simulink model "five_model"  (Simulink 7.9)
settings: Solver=ode3  StartTime=0.0  StopTime=5  FixedStep=0.005  RelTol=1e-3
values from neighbouring files (symbols this model uses):
  a = -1.0    (= -1)    [five_para.m]
  Ah = 0.234    [five_para.m]
  Ak = 0.227    [five_para.m]
  b = -2.0    (= -2)    [five_para.m]
  c = 0.23    [five_para.m]
  pf = 0.1786    [five_para.m]
  ph = 0.1786    [five_para.m]
  pw = 0.1786    [five_para.m]
  Ta = 0.38    [five_para.m]
  Tr = 0.04    [five_para.m]
  u0 = 0.1*rand(4,5)    [five_para.m]
  W = [0 -1 1 -1 -1; -1 0 -1 1 -1; 1 -1 0 -1 1; -1 1 -1 0 1;-1 -1 1 1 0]    [five_para.m]
settings Model: Creator=dede  LastModifiedBy=dede

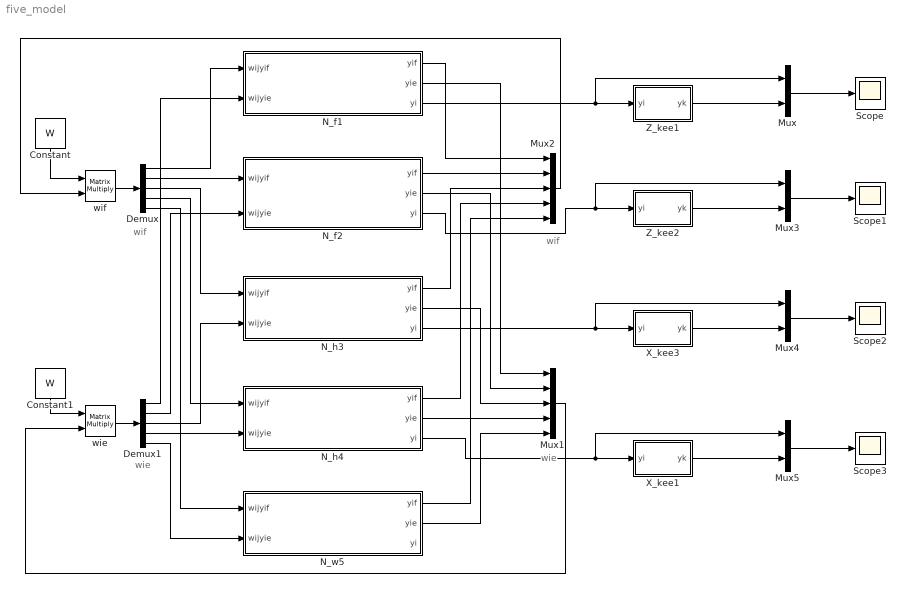
== system five_model ==
  note: wif
  note: wie
  note: wif
  note: wie
  Constant : Constant  Value=W
  Constant1 : Constant  Value=W
  Demux : Demux  Outputs=5
  Demux1 : Demux  Outputs=5
  Mux{,3..5} (4 alike) : Mux  Inputs=2
  Mux1 : Mux  Inputs=5
  Mux2 : Mux  Inputs=5
  N_f1 : Subsystem
  N_f2 : Subsystem
  N_h3 : Subsystem
  N_h4 : Subsystem
  N_w5 : Subsystem
  Scope{,1..3} (4 alike) : Scope
      Scope2 settings: SaveName=ScopeData2
      Scope3 settings: SaveName=ScopeData3
  X_kee1 : Subsystem
  X_kee3 : Subsystem
  Z_kee1 : Subsystem
  Z_kee2 : Subsystem
  wie : Product  Multiplication=Matrix(*)  RndMeth=Zero
  wif : Product  Multiplication=Matrix(*)  RndMeth=Zero
  wires:
  N_f1/1(yif) -> Mux2/1
  N_f2/1(yif) -> Mux2/2
  N_h3/1(yif) -> Mux2/3
  N_h4/1(yif) -> Mux2/4
  N_w5/1(yif) -> Mux2/5
  N_f1/2(yie) -> Mux1/1
  N_f2/2(yie) -> Mux1/2
  N_h3/2(yie) -> Mux1/3
  N_h4/2(yie) -> Mux1/4
  N_w5/2(yie) -> Mux1/5
  Demux/1 -> N_f1/1(wijyif)
  Demux/2 -> N_f2/1(wijyif)
  Demux/3 -> N_h3/1(wijyif)
  Demux/4 -> N_h4/1(wijyif)
  Demux/5 -> N_w5/1(wijyif)
  Demux1/1 -> N_f1/2(wijyie)
  Demux1/2 -> N_f2/2(wijyie)
  Demux1/3 -> N_h3/2(wijyie)
  Demux1/4 -> N_h4/2(wijyie)
  Demux1/5 -> N_w5/2(wijyie)
  Mux2/1 -> wif/2
  Constant/1 -> wif/1
  Mux1/1 -> wie/2
  Constant1/1 -> wie/1
  wie/1 -> Demux1/1
  wif/1 -> Demux/1
  N_f1/3(yi) -> Z_kee1/1(yi), Mux/1
  N_f2/3(yi) -> Z_kee2/1(yi), Mux3/1
  N_h3/3(yi) -> X_kee3/1(yi), Mux4/1
  N_h4/3(yi) -> X_kee1/1(yi), Mux5/1
  Z_kee1/1(yk) -> Mux/2
  Mux/1 -> Scope/1
  Z_kee2/1(yk) -> Mux3/2
  Mux3/1 -> Scope1/1
  X_kee3/1(yk) -> Mux4/2
  Mux4/1 -> Scope2/1
  Mux5/1 -> Scope3/1
  X_kee1/1(yk) -> Mux5/2

== system five_model/N_f1 ==
  wijyif : Inport
  wijyie : Inport  Port=2
  Gain : Gain  Gain=pf
  N_e1 : Subsystem
  N_f1 : Subsystem
  Sum : Sum  Inputs=+-
  yif : Outport
  yie : Outport  Port=2
  yi : Outport  Port=3
  wires:
  N_f1/2(yif) -> N_e1/1(yif), yif/1
  N_e1/2(yie) -> N_f1/1(yie), yie/1
  wijyif/1 -> N_f1/2(wijyif)
  wijyie/1 -> N_e1/2(wijyie)
  N_f1/1(uif) -> Sum/1
  N_e1/1(uie) -> Sum/2
  Sum/1 -> Gain/1
  Gain/1 -> yi/1

== system five_model/N_f2 ==
  wijyif : Inport
  wijyie : Inport  Port=2
  Gain : Gain  Gain=pf
  N_e1 : Subsystem
  N_f1 : Subsystem
  Sum : Sum  Inputs=+-
  yif : Outport
  yie : Outport  Port=2
  yi : Outport  Port=3
  wires:
  Gain/1 -> yi/1
  Sum/1 -> Gain/1
  N_e1/1(uie) -> Sum/2
  N_f1/1(uif) -> Sum/1
  wijyie/1 -> N_e1/2(wijyie)
  wijyif/1 -> N_f1/2(wijyif)
  N_e1/2(yie) -> yie/1, N_f1/1(yie)
  N_f1/2(yif) -> yif/1, N_e1/1(yif)

== system five_model/N_h3 ==
  wijyif : Inport
  wijyie : Inport  Port=2
  Gain : Gain  Gain=ph
  N_e1 : Subsystem
  N_f1 : Subsystem
  Sum : Sum  Inputs=+-
  yif : Outport
  yie : Outport  Port=2
  yi : Outport  Port=3
  wires:
  N_f1/2(yif) -> N_e1/1(yif), yif/1
  N_e1/2(yie) -> N_f1/1(yie), yie/1
  wijyif/1 -> N_f1/2(wijyif)
  wijyie/1 -> N_e1/2(wijyie)
  N_f1/1(uif) -> Sum/1
  N_e1/1(uie) -> Sum/2
  Sum/1 -> Gain/1
  Gain/1 -> yi/1

== system five_model/N_h4 ==
  wijyif : Inport
  wijyie : Inport  Port=2
  Gain : Gain  Gain=ph
  N_e1 : Subsystem
  N_f1 : Subsystem
  Sum : Sum  Inputs=+-
  yif : Outport
  yie : Outport  Port=2
  yi : Outport  Port=3
  wires:
  Gain/1 -> yi/1
  Sum/1 -> Gain/1
  N_e1/1(uie) -> Sum/2
  N_f1/1(uif) -> Sum/1
  wijyie/1 -> N_e1/2(wijyie)
  wijyif/1 -> N_f1/2(wijyif)
  N_e1/2(yie) -> yie/1, N_f1/1(yie)
  N_f1/2(yif) -> yif/1, N_e1/1(yif)

== system five_model/N_w5 ==
  wijyif : Inport
  wijyie : Inport  Port=2
  Gain : Gain  Gain=pw
  N_e1 : Subsystem
  N_f1 : Subsystem
  Sum : Sum  Inputs=+-
  yif : Outport
  yie : Outport  Port=2
  yi : Outport  Port=3
  wires:
  N_f1/2(yif) -> N_e1/1(yif), yif/1
  N_e1/2(yie) -> N_f1/1(yie), yie/1
  wijyif/1 -> N_f1/2(wijyif)
  wijyie/1 -> N_e1/2(wijyie)
  N_f1/1(uif) -> Sum/1
  N_e1/1(uie) -> Sum/2
  Sum/1 -> Gain/1
  Gain/1 -> yi/1

== system five_model/X_kee1 ==
  yi : Inport
  Constant2 : Constant  Value=0
  Derivative : Derivative
  Subsystem : Subsystem
  Switch : Switch
  yk : Outport
  wires:
  Switch/1 -> yk/1
  Subsystem/1(Out1) -> Switch/1
  Derivative/1 -> Switch/2
  yi/1 -> Subsystem/1(In1), Derivative/1
  Constant2/1 -> Switch/3

== system five_model/X_kee3 ==
  yi : Inport
  Constant2 : Constant  Value=0
  Derivative : Derivative
  Subsystem : Subsystem
  Switch : Switch
  yk : Outport
  wires:
  Constant2/1 -> Switch/3
  yi/1 -> Derivative/1, Subsystem/1(In1)
  Derivative/1 -> Switch/2
  Subsystem/1(Out1) -> Switch/1
  Switch/1 -> yk/1

== system five_model/Z_kee1 ==
  yi : Inport
  Constant2 : Constant  Value=0
  Derivative : Derivative
  Subsystem : Subsystem
  Switch : Switch
  yk : Outport
  wires:
  Constant2/1 -> Switch/3
  yi/1 -> Derivative/1, Subsystem/1(In1)
  Derivative/1 -> Switch/2
  Subsystem/1(Out1) -> Switch/1
  Switch/1 -> yk/1

== system five_model/Z_kee2 ==
  yi : Inport
  Constant2 : Constant  Value=0
  Derivative : Derivative
  Subsystem : Subsystem
  Switch : Switch
  yk : Outport
  wires:
  Switch/1 -> yk/1
  Subsystem/1(Out1) -> Switch/1
  Derivative/1 -> Switch/2
  yi/1 -> Subsystem/1(In1), Derivative/1
  Constant2/1 -> Switch/3

== system five_model/N_f1/N_e1 ==
  yif : Inport
  wijyie : Inport  Port=2
  Constant : Constant  Value=0
  uie0 : Subsystem
  vie : Subsystem
  yie0 : Switch
  uie : Outport
  yie : Outport  Port=2
  wires:
  vie/1(vie) -> uie0/1(vie)
  yif/1 -> uie0/2(yif)
  wijyie/1 -> uie0/3(wijyie)
  Constant/1 -> yie0/3
  uie0/1(uie) -> yie0/1, yie0/2, uie/1
  yie0/1 -> vie/1(yie), yie/1

== system five_model/N_f1/N_f1 ==
  yie : Inport
  wijyif : Inport  Port=2
  Constant : Constant  Value=0
  uif0 : Subsystem
  vif : Subsystem
  yif0 : Switch
  uif : Outport
  yif : Outport  Port=2
  wires:
  vif/1(vif) -> uif0/1(vif)
  Constant/1 -> yif0/3
  uif0/1(uif) -> yif0/1, yif0/2, uif/1
  yif0/1 -> vif/1(yif1), yif/1
  yie/1 -> uif0/2(yie)
  wijyif/1 -> uif0/3(wijyif)

== system five_model/N_f2/N_e1 ==
  yif : Inport
  wijyie : Inport  Port=2
  Constant : Constant  Value=0
  uie0 : Subsystem
  vie : Subsystem
  yie0 : Switch
  uie : Outport
  yie : Outport  Port=2
  wires:
  yie0/1 -> yie/1, vie/1(yie)
  uie0/1(uie) -> uie/1, yie0/2, yie0/1
  Constant/1 -> yie0/3
  wijyie/1 -> uie0/3(wijyie)
  yif/1 -> uie0/2(yif)
  vie/1(vie) -> uie0/1(vie)

== system five_model/N_f2/N_f1 ==
  yie : Inport
  wijyif : Inport  Port=2
  Constant : Constant  Value=0
  uif0 : Subsystem
  vif : Subsystem
  yif0 : Switch
  uif : Outport
  yif : Outport  Port=2
  wires:
  wijyif/1 -> uif0/3(wijyif)
  yie/1 -> uif0/2(yie)
  yif0/1 -> yif/1, vif/1(yif1)
  uif0/1(uif) -> uif/1, yif0/2, yif0/1
  Constant/1 -> yif0/3
  vif/1(vif) -> uif0/1(vif)

== system five_model/N_h3/N_e1 ==
  yif : Inport
  wijyie : Inport  Port=2
  Constant : Constant  Value=0
  uie0 : Subsystem
  vie : Subsystem
  yie0 : Switch
  uie : Outport
  yie : Outport  Port=2
  wires:
  vie/1(vie) -> uie0/1(vie)
  yif/1 -> uie0/2(yif)
  wijyie/1 -> uie0/3(wijyie)
  Constant/1 -> yie0/3
  uie0/1(uie) -> yie0/1, yie0/2, uie/1
  yie0/1 -> vie/1(yie), yie/1

== system five_model/N_h3/N_f1 ==
  yie : Inport
  wijyif : Inport  Port=2
  Constant : Constant  Value=0
  uif0 : Subsystem
  vif : Subsystem
  yif0 : Switch
  uif : Outport
  yif : Outport  Port=2
  wires:
  vif/1(vif) -> uif0/1(vif)
  Constant/1 -> yif0/3
  uif0/1(uif) -> yif0/1, yif0/2, uif/1
  yif0/1 -> vif/1(yif1), yif/1
  yie/1 -> uif0/2(yie)
  wijyif/1 -> uif0/3(wijyif)

== system five_model/N_h4/N_e1 ==
  yif : Inport
  wijyie : Inport  Port=2
  Constant : Constant  Value=0
  uie0 : Subsystem
  vie : Subsystem
  yie0 : Switch
  uie : Outport
  yie : Outport  Port=2
  wires:
  yie0/1 -> yie/1, vie/1(yie)
  uie0/1(uie) -> uie/1, yie0/2, yie0/1
  Constant/1 -> yie0/3
  wijyie/1 -> uie0/3(wijyie)
  yif/1 -> uie0/2(yif)
  vie/1(vie) -> uie0/1(vie)

== system five_model/N_h4/N_f1 ==
  yie : Inport
  wijyif : Inport  Port=2
  Constant : Constant  Value=0
  uif0 : Subsystem
  vif : Subsystem
  yif0 : Switch
  uif : Outport
  yif : Outport  Port=2
  wires:
  wijyif/1 -> uif0/3(wijyif)
  yie/1 -> uif0/2(yie)
  yif0/1 -> yif/1, vif/1(yif1)
  uif0/1(uif) -> uif/1, yif0/2, yif0/1
  Constant/1 -> yif0/3
  vif/1(vif) -> uif0/1(vif)

== system five_model/N_w5/N_e1 ==
  yif : Inport
  wijyie : Inport  Port=2
  Constant : Constant  Value=0
  uie0 : Subsystem
  vie : Subsystem
  yie0 : Switch
  uie : Outport
  yie : Outport  Port=2
  wires:
  vie/1(vie) -> uie0/1(vie)
  yif/1 -> uie0/2(yif)
  wijyie/1 -> uie0/3(wijyie)
  Constant/1 -> yie0/3
  uie0/1(uie) -> yie0/1, yie0/2, uie/1
  yie0/1 -> vie/1(yie), yie/1

== system five_model/N_w5/N_f1 ==
  yie : Inport
  wijyif : Inport  Port=2
  Constant : Constant  Value=0
  uif0 : Subsystem
  vif : Subsystem
  yif0 : Switch
  uif : Outport
  yif : Outport  Port=2
  wires:
  vif/1(vif) -> uif0/1(vif)
  Constant/1 -> yif0/3
  uif0/1(uif) -> yif0/1, yif0/2, uif/1
  yif0/1 -> vif/1(yif1), yif/1
  yie/1 -> uif0/2(yie)
  wijyif/1 -> uif0/3(wijyif)

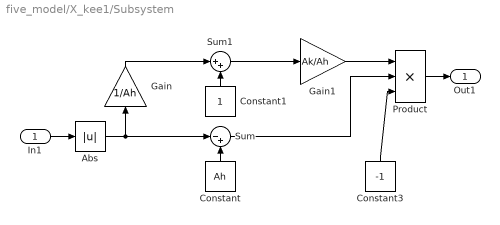
== system five_model/X_kee1/Subsystem ==
  In1 : Inport
  Abs : Abs
  Constant : Constant  Value=Ah
  Constant1 : Constant
  Constant3 : Constant  Value=-1
  Gain : Gain  Gain=1/Ah
  Gain1 : Gain  Gain=Ak/Ah
  Product : Product  Inputs=3  RndMeth=Zero
  Sum : Sum  Inputs=|-+
  Sum1 : Sum  Inputs=|++
  Out1 : Outport
  wires:
  In1/1 -> Abs/1
  Product/1 -> Out1/1
  Constant3/1 -> Product/3
  Gain1/1 -> Product/1
  Sum/1 -> Product/2
  Sum1/1 -> Gain1/1
  Gain/1 -> Sum1/1
  Constant1/1 -> Sum1/2
  Constant/1 -> Sum/2
  Abs/1 -> Gain/1, Sum/1

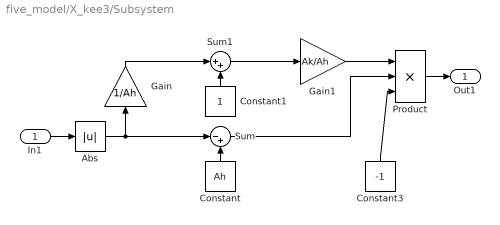
== system five_model/X_kee3/Subsystem ==
  In1 : Inport
  Abs : Abs
  Constant : Constant  Value=Ah
  Constant1 : Constant
  Constant3 : Constant  Value=-1
  Gain : Gain  Gain=1/Ah
  Gain1 : Gain  Gain=Ak/Ah
  Product : Product  Inputs=3  RndMeth=Zero
  Sum : Sum  Inputs=|-+
  Sum1 : Sum  Inputs=|++
  Out1 : Outport
  wires:
  Abs/1 -> Sum/1, Gain/1
  Constant/1 -> Sum/2
  Constant1/1 -> Sum1/2
  Gain/1 -> Sum1/1
  Sum1/1 -> Gain1/1
  Sum/1 -> Product/2
  Gain1/1 -> Product/1
  Constant3/1 -> Product/3
  Product/1 -> Out1/1
  In1/1 -> Abs/1

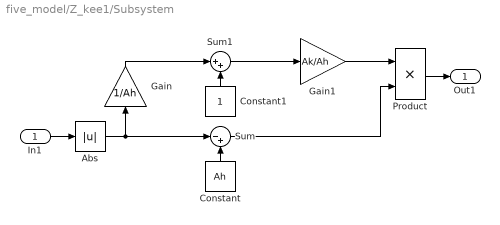
== system five_model/Z_kee1/Subsystem ==
  In1 : Inport
  Abs : Abs
  Constant : Constant  Value=Ah
  Constant1 : Constant
  Gain : Gain  Gain=1/Ah
  Gain1 : Gain  Gain=Ak/Ah
  Product : Product  RndMeth=Zero
  Sum : Sum  Inputs=|-+
  Sum1 : Sum  Inputs=|++
  Out1 : Outport
  wires:
  Abs/1 -> Sum/1, Gain/1
  Constant/1 -> Sum/2
  Constant1/1 -> Sum1/2
  Gain/1 -> Sum1/1
  Sum1/1 -> Gain1/1
  Sum/1 -> Product/2
  Gain1/1 -> Product/1
  Product/1 -> Out1/1
  In1/1 -> Abs/1

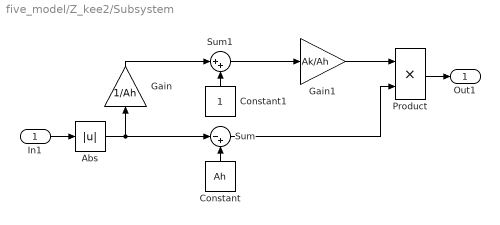
== system five_model/Z_kee2/Subsystem ==
  In1 : Inport
  Abs : Abs
  Constant : Constant  Value=Ah
  Constant1 : Constant
  Gain : Gain  Gain=1/Ah
  Gain1 : Gain  Gain=Ak/Ah
  Product : Product  RndMeth=Zero
  Sum : Sum  Inputs=|-+
  Sum1 : Sum  Inputs=|++
  Out1 : Outport
  wires:
  In1/1 -> Abs/1
  Product/1 -> Out1/1
  Gain1/1 -> Product/1
  Sum/1 -> Product/2
  Sum1/1 -> Gain1/1
  Gain/1 -> Sum1/1
  Constant1/1 -> Sum1/2
  Constant/1 -> Sum/2
  Abs/1 -> Gain/1, Sum/1

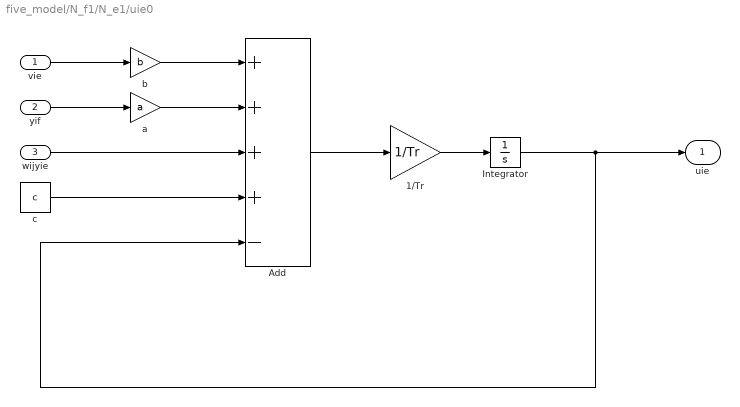
== system five_model/N_f1/N_e1/uie0 ==
  vie : Inport
  yif : Inport  Port=2
  wijyie : Inport  Port=3
  1/Tr : Gain  Gain=1/Tr
  Add : Sum  Inputs=++++-
  Integrator : Integrator  InitialCondition=u0(3,1)
  a : Gain  Gain=a
  b : Gain  Gain=b
  c : Constant  Value=c
  uie : Outport
  wires:
  vie/1 -> b/1
  b/1 -> Add/1
  yif/1 -> a/1
  a/1 -> Add/2
  wijyie/1 -> Add/3
  c/1 -> Add/4
  Add/1 -> 1/Tr/1
  1/Tr/1 -> Integrator/1
  Integrator/1 -> Add/5, uie/1

== system five_model/N_f1/N_e1/vie ==
  yie : Inport
  1/Ta : Gain  Gain=1/Ta
  1/Ta1 : Gain  Gain=1/Ta
  Add : Sum  Inputs=+-
  Integrator : Integrator  InitialCondition=u0(4,1)
  vie : Outport
  wires:
  yie/1 -> 1/Ta/1
  1/Ta/1 -> Add/1
  Add/1 -> Integrator/1
  Integrator/1 -> 1/Ta1/1, vie/1
  1/Ta1/1 -> Add/2

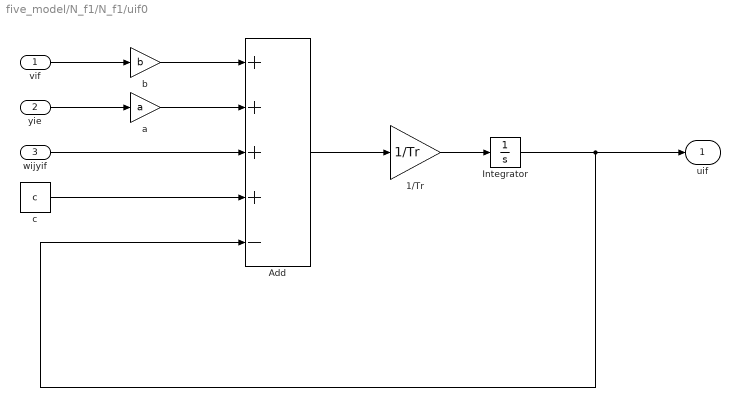
== system five_model/N_f1/N_f1/uif0 ==
  vif : Inport
  yie : Inport  Port=2
  wijyif : Inport  Port=3
  1/Tr : Gain  Gain=1/Tr
  Add : Sum  Inputs=++++-
  Integrator : Integrator  InitialCondition=u0(1,1)
  a : Gain  Gain=a
  b : Gain  Gain=b
  c : Constant  Value=c
  uif : Outport
  wires:
  vif/1 -> b/1
  b/1 -> Add/1
  yie/1 -> a/1
  a/1 -> Add/2
  wijyif/1 -> Add/3
  c/1 -> Add/4
  Add/1 -> 1/Tr/1
  1/Tr/1 -> Integrator/1
  Integrator/1 -> Add/5, uif/1

== system five_model/N_f1/N_f1/vif ==
  yif1 : Inport
  1/Ta : Gain  Gain=1/Ta
  1/Ta1 : Gain  Gain=1/Ta
  Add : Sum  Inputs=+-
  Integrator : Integrator  InitialCondition=u0(2,1)
  vif : Outport
  wires:
  yif1/1 -> 1/Ta/1
  1/Ta/1 -> Add/1
  Add/1 -> Integrator/1
  Integrator/1 -> 1/Ta1/1, vif/1
  1/Ta1/1 -> Add/2

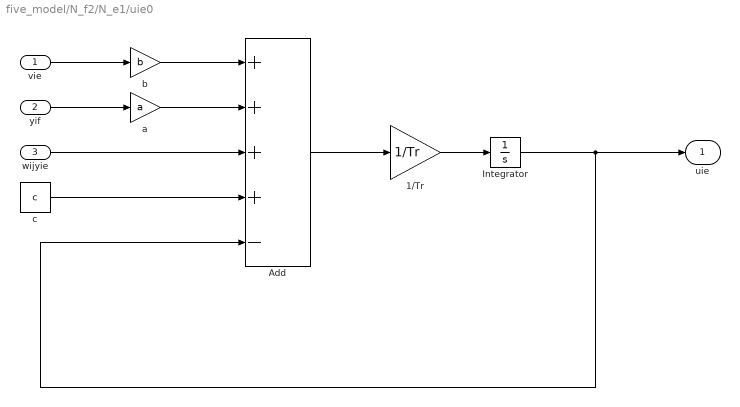
== system five_model/N_f2/N_e1/uie0 ==
  vie : Inport
  yif : Inport  Port=2
  wijyie : Inport  Port=3
  1/Tr : Gain  Gain=1/Tr
  Add : Sum  Inputs=++++-
  Integrator : Integrator  InitialCondition=u0(3,2)
  a : Gain  Gain=a
  b : Gain  Gain=b
  c : Constant  Value=c
  uie : Outport
  wires:
  Integrator/1 -> uie/1, Add/5
  1/Tr/1 -> Integrator/1
  Add/1 -> 1/Tr/1
  c/1 -> Add/4
  wijyie/1 -> Add/3
  a/1 -> Add/2
  yif/1 -> a/1
  b/1 -> Add/1
  vie/1 -> b/1

== system five_model/N_f2/N_e1/vie ==
  yie : Inport
  1/Ta : Gain  Gain=1/Ta
  1/Ta1 : Gain  Gain=1/Ta
  Add : Sum  Inputs=+-
  Integrator : Integrator  InitialCondition=u0(4,2)
  vie : Outport
  wires:
  1/Ta1/1 -> Add/2
  Integrator/1 -> vie/1, 1/Ta1/1
  Add/1 -> Integrator/1
  1/Ta/1 -> Add/1
  yie/1 -> 1/Ta/1

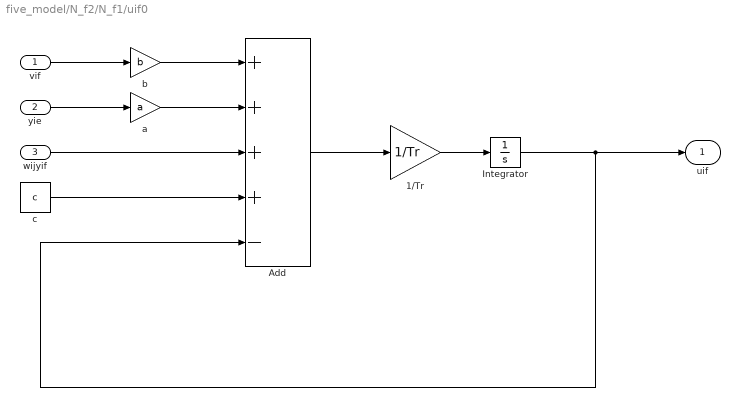
== system five_model/N_f2/N_f1/uif0 ==
  vif : Inport
  yie : Inport  Port=2
  wijyif : Inport  Port=3
  1/Tr : Gain  Gain=1/Tr
  Add : Sum  Inputs=++++-
  Integrator : Integrator  InitialCondition=u0(2,1)
  a : Gain  Gain=a
  b : Gain  Gain=b
  c : Constant  Value=c
  uif : Outport
  wires:
  Integrator/1 -> uif/1, Add/5
  1/Tr/1 -> Integrator/1
  Add/1 -> 1/Tr/1
  c/1 -> Add/4
  wijyif/1 -> Add/3
  a/1 -> Add/2
  yie/1 -> a/1
  b/1 -> Add/1
  vif/1 -> b/1

== system five_model/N_f2/N_f1/vif ==
  yif1 : Inport
  1/Ta : Gain  Gain=1/Ta
  1/Ta1 : Gain  Gain=1/Ta
  Add : Sum  Inputs=+-
  Integrator : Integrator  InitialCondition=u0(2,2)
  vif : Outport
  wires:
  1/Ta1/1 -> Add/2
  Integrator/1 -> vif/1, 1/Ta1/1
  Add/1 -> Integrator/1
  1/Ta/1 -> Add/1
  yif1/1 -> 1/Ta/1

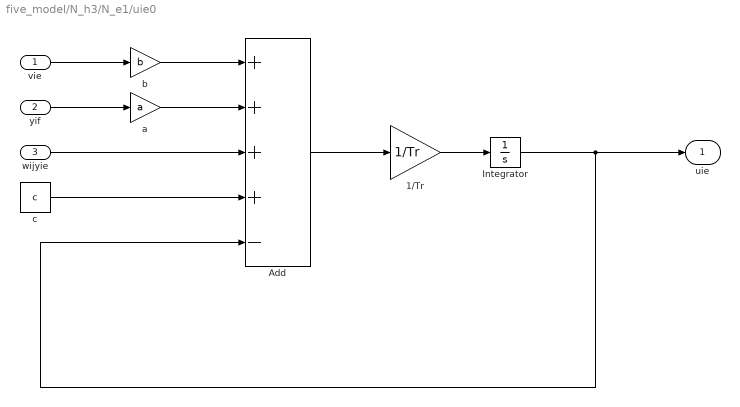
== system five_model/N_h3/N_e1/uie0 ==
  vie : Inport
  yif : Inport  Port=2
  wijyie : Inport  Port=3
  1/Tr : Gain  Gain=1/Tr
  Add : Sum  Inputs=++++-
  Integrator : Integrator  InitialCondition=u0(3,3)
  a : Gain  Gain=a
  b : Gain  Gain=b
  c : Constant  Value=c
  uie : Outport
  wires:
  vie/1 -> b/1
  b/1 -> Add/1
  yif/1 -> a/1
  a/1 -> Add/2
  wijyie/1 -> Add/3
  c/1 -> Add/4
  Add/1 -> 1/Tr/1
  1/Tr/1 -> Integrator/1
  Integrator/1 -> Add/5, uie/1

== system five_model/N_h3/N_e1/vie ==
  yie : Inport
  1/Ta : Gain  Gain=1/Ta
  1/Ta1 : Gain  Gain=1/Ta
  Add : Sum  Inputs=+-
  Integrator : Integrator  InitialCondition=u0(4,3)
  vie : Outport
  wires:
  yie/1 -> 1/Ta/1
  1/Ta/1 -> Add/1
  Add/1 -> Integrator/1
  Integrator/1 -> 1/Ta1/1, vie/1
  1/Ta1/1 -> Add/2

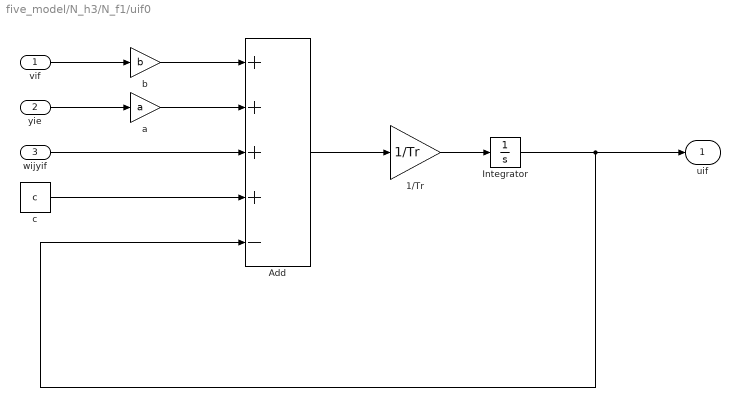
== system five_model/N_h3/N_f1/uif0 ==
  vif : Inport
  yie : Inport  Port=2
  wijyif : Inport  Port=3
  1/Tr : Gain  Gain=1/Tr
  Add : Sum  Inputs=++++-
  Integrator : Integrator  InitialCondition=u0(1,3)
  a : Gain  Gain=a
  b : Gain  Gain=b
  c : Constant  Value=c
  uif : Outport
  wires:
  vif/1 -> b/1
  b/1 -> Add/1
  yie/1 -> a/1
  a/1 -> Add/2
  wijyif/1 -> Add/3
  c/1 -> Add/4
  Add/1 -> 1/Tr/1
  1/Tr/1 -> Integrator/1
  Integrator/1 -> Add/5, uif/1

== system five_model/N_h3/N_f1/vif ==
  yif1 : Inport
  1/Ta : Gain  Gain=1/Ta
  1/Ta1 : Gain  Gain=1/Ta
  Add : Sum  Inputs=+-
  Integrator : Integrator  InitialCondition=u0(2,3)
  vif : Outport
  wires:
  yif1/1 -> 1/Ta/1
  1/Ta/1 -> Add/1
  Add/1 -> Integrator/1
  Integrator/1 -> 1/Ta1/1, vif/1
  1/Ta1/1 -> Add/2

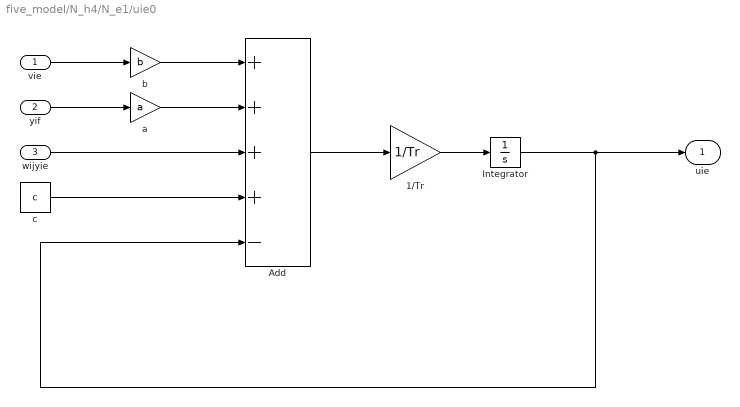
== system five_model/N_h4/N_e1/uie0 ==
  vie : Inport
  yif : Inport  Port=2
  wijyie : Inport  Port=3
  1/Tr : Gain  Gain=1/Tr
  Add : Sum  Inputs=++++-
  Integrator : Integrator  InitialCondition=u0(3,4)
  a : Gain  Gain=a
  b : Gain  Gain=b
  c : Constant  Value=c
  uie : Outport
  wires:
  Integrator/1 -> uie/1, Add/5
  1/Tr/1 -> Integrator/1
  Add/1 -> 1/Tr/1
  c/1 -> Add/4
  wijyie/1 -> Add/3
  a/1 -> Add/2
  yif/1 -> a/1
  b/1 -> Add/1
  vie/1 -> b/1

== system five_model/N_h4/N_e1/vie ==
  yie : Inport
  1/Ta : Gain  Gain=1/Ta
  1/Ta1 : Gain  Gain=1/Ta
  Add : Sum  Inputs=+-
  Integrator : Integrator  InitialCondition=u0(4,4)
  vie : Outport
  wires:
  1/Ta1/1 -> Add/2
  Integrator/1 -> vie/1, 1/Ta1/1
  Add/1 -> Integrator/1
  1/Ta/1 -> Add/1
  yie/1 -> 1/Ta/1

== system five_model/N_h4/N_f1/uif0 ==
  vif : Inport
  yie : Inport  Port=2
  wijyif : Inport  Port=3
  1/Tr : Gain  Gain=1/Tr
  Add : Sum  Inputs=++++-
  Integrator : Integrator  InitialCondition=u0(1,4)
  a : Gain  Gain=a
  b : Gain  Gain=b
  c : Constant  Value=c
  uif : Outport
  wires:
  Integrator/1 -> uif/1, Add/5
  1/Tr/1 -> Integrator/1
  Add/1 -> 1/Tr/1
  c/1 -> Add/4
  wijyif/1 -> Add/3
  a/1 -> Add/2
  yie/1 -> a/1
  b/1 -> Add/1
  vif/1 -> b/1

== system five_model/N_h4/N_f1/vif ==
  yif1 : Inport
  1/Ta : Gain  Gain=1/Ta
  1/Ta1 : Gain  Gain=1/Ta
  Add : Sum  Inputs=+-
  Integrator : Integrator  InitialCondition=u0(2,4)
  vif : Outport
  wires:
  1/Ta1/1 -> Add/2
  Integrator/1 -> vif/1, 1/Ta1/1
  Add/1 -> Integrator/1
  1/Ta/1 -> Add/1
  yif1/1 -> 1/Ta/1

== system five_model/N_w5/N_e1/uie0 ==
  vie : Inport
  yif : Inport  Port=2
  wijyie : Inport  Port=3
  1/Tr : Gain  Gain=1/Tr
  Add : Sum  Inputs=++++-
  Integrator : Integrator  InitialCondition=u0(3,5)
  a : Gain  Gain=a
  b : Gain  Gain=b
  c : Constant  Value=c
  uie : Outport
  wires:
  vie/1 -> b/1
  b/1 -> Add/1
  yif/1 -> a/1
  a/1 -> Add/2
  wijyie/1 -> Add/3
  c/1 -> Add/4
  Add/1 -> 1/Tr/1
  1/Tr/1 -> Integrator/1
  Integrator/1 -> Add/5, uie/1

== system five_model/N_w5/N_e1/vie ==
  yie : Inport
  1/Ta : Gain  Gain=1/Ta
  1/Ta1 : Gain  Gain=1/Ta
  Add : Sum  Inputs=+-
  Integrator : Integrator  InitialCondition=u0(4,5)
  vie : Outport
  wires:
  yie/1 -> 1/Ta/1
  1/Ta/1 -> Add/1
  Add/1 -> Integrator/1
  Integrator/1 -> 1/Ta1/1, vie/1
  1/Ta1/1 -> Add/2

== system five_model/N_w5/N_f1/uif0 ==
  vif : Inport
  yie : Inport  Port=2
  wijyif : Inport  Port=3
  1/Tr : Gain  Gain=1/Tr
  Add : Sum  Inputs=++++-
  Integrator : Integrator  InitialCondition=u0(1,5)
  a : Gain  Gain=a
  b : Gain  Gain=b
  c : Constant  Value=c
  uif : Outport
  wires:
  vif/1 -> b/1
  b/1 -> Add/1
  yie/1 -> a/1
  a/1 -> Add/2
  wijyif/1 -> Add/3
  c/1 -> Add/4
  Add/1 -> 1/Tr/1
  1/Tr/1 -> Integrator/1
  Integrator/1 -> Add/5, uif/1

== system five_model/N_w5/N_f1/vif ==
  yif1 : Inport
  1/Ta : Gain  Gain=1/Ta
  1/Ta1 : Gain  Gain=1/Ta
  Add : Sum  Inputs=+-
  Integrator : Integrator  InitialCondition=u0(2,5)
  vif : Outport
  wires:
  yif1/1 -> 1/Ta/1
  1/Ta/1 -> Add/1
  Add/1 -> Integrator/1
  Integrator/1 -> 1/Ta1/1, vif/1
  1/Ta1/1 -> Add/2
